simulink model "estf_freqest_withEV"  (R2021a)
settings: Solver=VariableStepAuto  StartTime=0.0  StopTime=3  RelTol=1e-3
undefined symbols (not defined in the file or in its folder): Ion, Lithium
libraries: spsCurrentMeasurementLib x25, spsVoltageMeasurementLib x19, spsSeriesRLCBranchLib x11, spsGroundLib x6, powerlib_extras x5, dspsigops x3, spsPower3phInstantaneousLib x3, eeTotalHarmonicDistorsion x3, spsIGBTDiodeLib x2, spsUniversalBridgeLib x2, spsThreePhaseSourceLib x1, spsBatteryLib x1
(part 2 of 2)

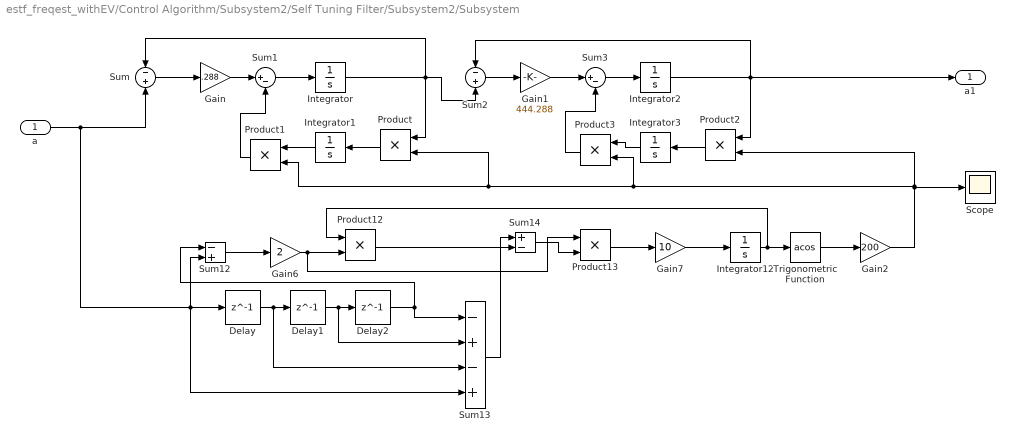
== system estf_freqest_withEV/Control Algorithm/Subsystem2/Self Tuning Filter/Subsystem2/Subsystem ==
  a : Inport
  Delay : Delay  DelayLength=1
  Delay1 : Delay  DelayLength=1
  Delay2 : Delay  DelayLength=1
  Gain : Gain  Gain=.288
  Gain1 : Gain  Gain=444.288
  Gain2 : Gain  Gain=200
  Gain6 : Gain  Gain=2
  Gain7 : Gain  Gain=10
  Integrator{,1..3,12} (5 alike) : Integrator
  Product{,1..3,12..13} (6 alike) : Product
  Scope : Scope
  Sum : Sum  Inputs=-+
  Sum1 : Sum  Inputs=|+-
  Sum12 : Sum  Inputs=-+
  Sum13 : Sum  Inputs=-+-+
  Sum14 : Sum  Inputs=+-
  Sum2 : Sum  Inputs=-+
  Sum3 : Sum  Inputs=|+-
  Trigonometric Function : Trigonometry  Operator=acos
  a1 : Outport
  wires:
  Product13/1 -> Gain7/1
  Gain6/1 -> Product13/1, Product12/2
  Product12/1 -> Sum14/2
  Gain1/1 -> Sum3/1
  Product3/1 -> Sum3/2
  Gain7/1 -> Integrator12/1
  Sum14/1 -> Product13/2
  Sum/1 -> Gain/1
  Delay/1 -> Sum13/3, Delay1/1
  a/1 -> Sum13/4, Sum12/2, Delay/1, Sum/2
  Integrator/1 -> Sum/1, Sum2/2, Product/1
  Sum3/1 -> Integrator2/1
  Sum13/1 -> Sum14/1
  Gain/1 -> Sum1/1
  Integrator2/1 -> a1/1, Product2/1, Sum2/1
  Integrator3/1 -> Product3/1
  Sum12/1 -> Gain6/1
  Delay1/1 -> Sum13/2, Delay2/1
  Integrator1/1 -> Product1/1
  Sum1/1 -> Integrator/1
  Sum2/1 -> Gain1/1
  Product2/1 -> Integrator3/1
  Product/1 -> Integrator1/1
  Product1/1 -> Sum1/2
  Integrator12/1 -> Product12/1, Trigonometric Function/1
  Delay2/1 -> Sum13/1, Sum12/1
  Trigonometric Function/1 -> Gain2/1
  Gain2/1 -> Product2/2, Product1/2, Product/2, Product3/2, Scope/1

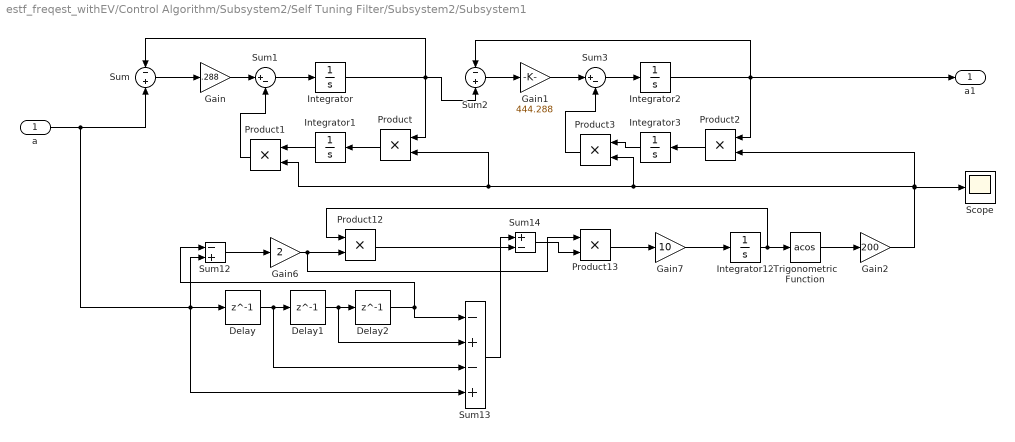
== system estf_freqest_withEV/Control Algorithm/Subsystem2/Self Tuning Filter/Subsystem2/Subsystem1 ==
  a : Inport
  Delay : Delay  DelayLength=1
  Delay1 : Delay  DelayLength=1
  Delay2 : Delay  DelayLength=1
  Gain : Gain  Gain=.288
  Gain1 : Gain  Gain=444.288
  Gain2 : Gain  Gain=200
  Gain6 : Gain  Gain=2
  Gain7 : Gain  Gain=10
  Integrator{,1..3,12} (5 alike) : Integrator
  Product{,1..3,12..13} (6 alike) : Product
  Scope : Scope
  Sum : Sum  Inputs=-+
  Sum1 : Sum  Inputs=|+-
  Sum12 : Sum  Inputs=-+
  Sum13 : Sum  Inputs=-+-+
  Sum14 : Sum  Inputs=+-
  Sum2 : Sum  Inputs=-+
  Sum3 : Sum  Inputs=|+-
  Trigonometric Function : Trigonometry  Operator=acos
  a1 : Outport
  wires:
  Product13/1 -> Gain7/1
  Gain6/1 -> Product13/1, Product12/2
  Product12/1 -> Sum14/2
  Gain1/1 -> Sum3/1
  Product3/1 -> Sum3/2
  Gain7/1 -> Integrator12/1
  Sum14/1 -> Product13/2
  Sum/1 -> Gain/1
  Delay/1 -> Sum13/3, Delay1/1
  a/1 -> Sum13/4, Sum12/2, Delay/1, Sum/2
  Integrator/1 -> Sum/1, Sum2/2, Product/1
  Sum3/1 -> Integrator2/1
  Sum13/1 -> Sum14/1
  Gain/1 -> Sum1/1
  Integrator2/1 -> a1/1, Product2/1, Sum2/1
  Integrator3/1 -> Product3/1
  Sum12/1 -> Gain6/1
  Delay1/1 -> Sum13/2, Delay2/1
  Integrator1/1 -> Product1/1
  Sum1/1 -> Integrator/1
  Sum2/1 -> Gain1/1
  Product2/1 -> Integrator3/1
  Product/1 -> Integrator1/1
  Product1/1 -> Sum1/2
  Integrator12/1 -> Product12/1, Trigonometric Function/1
  Delay2/1 -> Sum13/1, Sum12/1
  Trigonometric Function/1 -> Gain2/1
  Gain2/1 -> Product2/2, Product1/2, Product/2, Product3/2, Scope/1

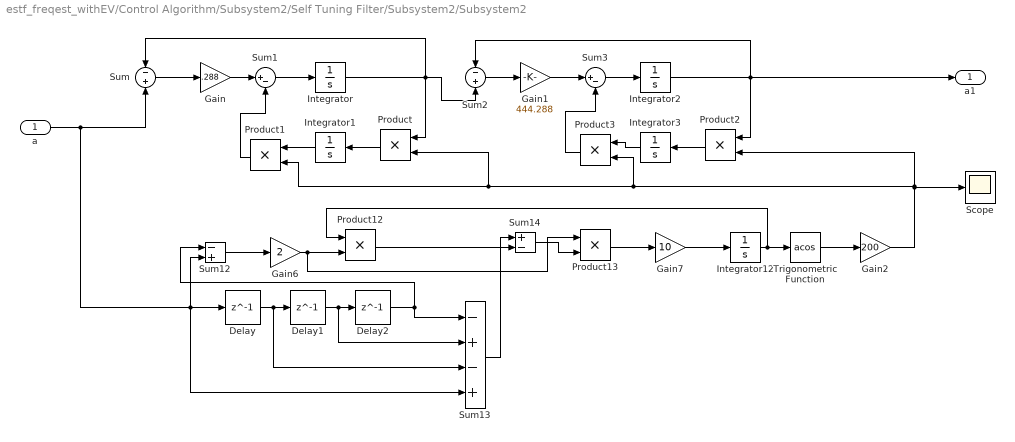
== system estf_freqest_withEV/Control Algorithm/Subsystem2/Self Tuning Filter/Subsystem2/Subsystem2 ==
  a : Inport
  Delay : Delay  DelayLength=1
  Delay1 : Delay  DelayLength=1
  Delay2 : Delay  DelayLength=1
  Gain : Gain  Gain=.288
  Gain1 : Gain  Gain=444.288
  Gain2 : Gain  Gain=200
  Gain6 : Gain  Gain=2
  Gain7 : Gain  Gain=10
  Integrator{,1..3,12} (5 alike) : Integrator
  Product{,1..3,12..13} (6 alike) : Product
  Scope : Scope
  Sum : Sum  Inputs=-+
  Sum1 : Sum  Inputs=|+-
  Sum12 : Sum  Inputs=-+
  Sum13 : Sum  Inputs=-+-+
  Sum14 : Sum  Inputs=+-
  Sum2 : Sum  Inputs=-+
  Sum3 : Sum  Inputs=|+-
  Trigonometric Function : Trigonometry  Operator=acos
  a1 : Outport
  wires:
  Product13/1 -> Gain7/1
  Gain6/1 -> Product13/1, Product12/2
  Product12/1 -> Sum14/2
  Gain1/1 -> Sum3/1
  Product3/1 -> Sum3/2
  Gain7/1 -> Integrator12/1
  Sum14/1 -> Product13/2
  Sum/1 -> Gain/1
  Delay/1 -> Sum13/3, Delay1/1
  a/1 -> Sum13/4, Sum12/2, Delay/1, Sum/2
  Integrator/1 -> Sum/1, Sum2/2, Product/1
  Sum3/1 -> Integrator2/1
  Sum13/1 -> Sum14/1
  Gain/1 -> Sum1/1
  Integrator2/1 -> a1/1, Product2/1, Sum2/1
  Integrator3/1 -> Product3/1
  Sum12/1 -> Gain6/1
  Delay1/1 -> Sum13/2, Delay2/1
  Integrator1/1 -> Product1/1
  Sum1/1 -> Integrator/1
  Sum2/1 -> Gain1/1
  Product2/1 -> Integrator3/1
  Product/1 -> Integrator1/1
  Product1/1 -> Sum1/2
  Integrator12/1 -> Product12/1, Trigonometric Function/1
  Delay2/1 -> Sum13/1, Sum12/1
  Trigonometric Function/1 -> Gain2/1
  Gain2/1 -> Product2/2, Product1/2, Product/2, Product3/2, Scope/1

== matlab function estf_freqest_withEV/MPPT ==
  settings: updateMethod=DISCRETE  sampleTime=1e-4
  data: tv input; Ipvin input; Vpvin input; Ipvin1 input; Vpvin1 input; Vdcref output; Vdcrefold input
function Vdcref = fcn(tv,Ipvin,Vpvin,Ipvin1,Vpvin1,Vdcrefold)
%#codegen
delVdc=0.2;
a=10;
delVpv=Vpvin-Vpvin1;
delIpv=Ipvin-Ipvin1;
if(tv>=0.6)
if(delVpv==0)
    if(delIpv==0)
        Vdcrefnew=Vdcrefold;
    else
        if(delIpv>0)
            Vdcrefnew=Vdcrefold-(delIpv/delVpv)*a;
    else
        Vdcrefnew=Vdcrefold+(delIpv/delVpv)*a;
        end
    end
    else
        if(delIpv/delVpv==-Ipvin/Vpvin)
            Vdcrefnew=Vdcrefold;
        else
            if(delIpv/delVpv>-Ipvin/Vpvin)
                Vdcrefnew=Vdcrefold-(delIpv/delVpv)*a;
            else
                Vdcrefnew=Vdcrefold+(delIpv/delVpv)*a;
            end
        end
end
Vdcref=Vdcrefnew;
else
Vdcref=810;
end


%Vdcref=658;
